simulink model "Part_E_a"  (R2016a)
settings: Solver=VariableStepAuto  StartTime=0.0  StopTime=20  RelTol=1e-3
values from neighbouring files (symbols this model uses):
  Ad = sysd.A    [Project_5.m]
  Ado = Ad-L*[1 0 0 0]    [Project_5.m]
  Bd = sysd.B    [Project_5.m]
  Bdo = [Bd L]    [Project_5.m]
  Cd = sysd.C    [Project_5.m]
  Dd = sysd.D    [Project_5.m]
  Kd = acker(Ad,Bd,[0,0,0,0])    [Project_5.m]
undefined symbols (not defined in the file or in its folder): DiscIntNeverNeededParam
libraries: simulink x1
settings Model: Creator=ACER  LastModifiedBy=ACER

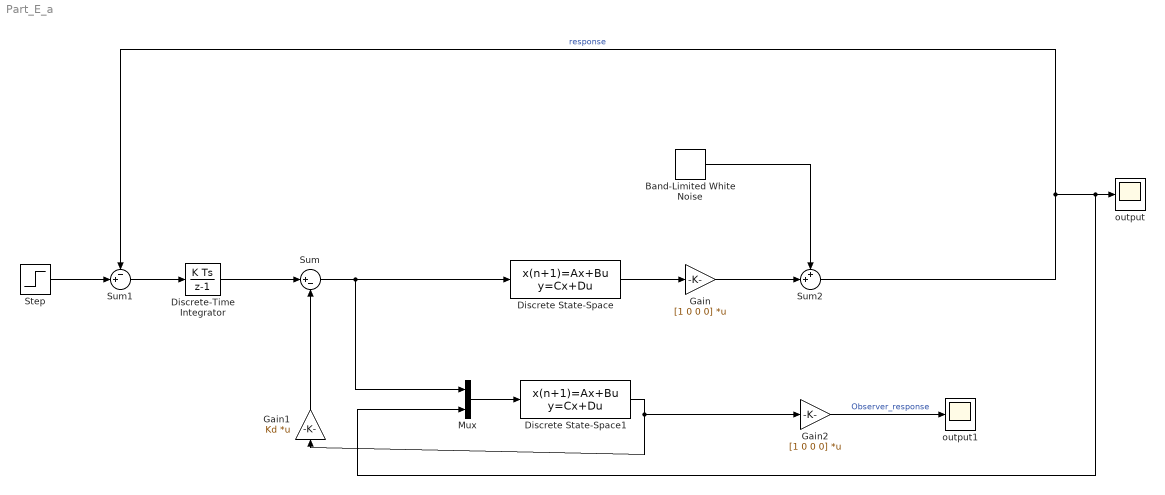
== system Part_E_a ==
  Band-Limited White Noise : simulink/Sources/Band-Limited White Noise  Cov=[0.1]  Ts=.5  seed=[23341]
  Discrete State-Space : DiscreteStateSpace  A=Ad  B=Bd  C=Cd  D=Dd  SampleTime=.5
  Discrete State-Space1 : DiscreteStateSpace  A=Ado  B=Bdo  C=Cd  D=[0 0;0 0;0 0;0 0]  SampleTime=.5
  Discrete-Time Integrator : DiscreteIntegrator  gainval=2.5560e+03  InitialConditionSetting=State (most efficient)  SampleTime=.5  ICPrevOutput=DiscIntNeverNeededParam  ICPrevScaledInput=DiscIntNeverNeededParam
  Gain : Gain  Gain=[1 0 0 0]  Multiplication=Matrix(K*u)
  Gain1 : Gain  Gain=Kd  Multiplication=Matrix(K*u)
  Gain2 : Gain  Gain=[1 0 0 0]  Multiplication=Matrix(K*u)
  Mux : Mux  Inputs=2
  Step : Step  SampleTime=0
  Sum : Sum  Inputs=|+-
  Sum1 : Sum  Inputs=-+|
  Sum2 : Sum  Inputs=++|
  output : Scope
  output1 : Scope
  wires:
  Sum/1 -> Mux/1, Discrete State-Space/1
  Discrete State-Space/1 -> Gain/1
  Mux/1 -> Discrete State-Space1/1
  Discrete State-Space1/1 -> Gain2/1, Gain1/1
  Gain1/1 -> Sum/2
  Discrete-Time Integrator/1 -> Sum/1
  Sum1/1 -> Discrete-Time Integrator/1
  Step/1 -> Sum1/2
  Gain2/1 -> output1/1  "Observer_response"
  Gain/1 -> Sum2/2
  Band-Limited White Noise/1 -> Sum2/1
  Sum2/1 -> Sum1/1, Mux/2, output/1  "response"
